simulink model "single-phase half bridge-controlled rectifier with resistive load"  (R2022a)
settings: Solver=VariableStepAuto  StartTime=0.0  StopTime=1  RelTol=1e-3
libraries: spsCurrentMeasurementLib x2, spsDiodeLib x2, spsSeriesRLCBranchLib x2, spsThyristorLib x2, spsVoltageMeasurementLib x2, spsACVoltageSourceLib x1, spspowerguiLib x1
settings Model: Creator=Joy  LastModifiedBy=Joy
settings SolverCC: AlgebraicLoopSolver=TrustRegion
settings DataIOCC: ReturnWorkspaceOutputs=off
settings RTWCC: DLArmComputeVersion=19.05

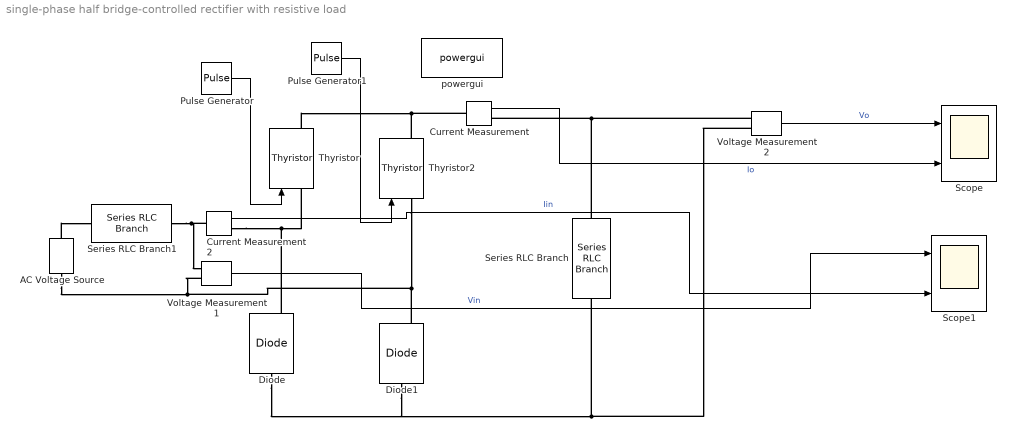
== system single-phase half bridge-controlled rectifier with resistive load ==
  AC Voltage Source : spsACVoltageSourceLib/AC Voltage Source  Amplitude=424.26  Phase=0  Frequency=60  SampleTime=0  Measurements=None  BusType=swing  Pref=10e3  Qref=0  Qmin=-inf  Qmax=+inf
  Current Measurement : spsCurrentMeasurementLib/Current Measurement  PhasorSimulation=off  OutputType=Complex  PSBequivalent=0
  Current Measurement2 : spsCurrentMeasurementLib/Current Measurement  PhasorSimulation=off  OutputType=Complex  PSBequivalent=0
  Diode : spsDiodeLib/Diode  Ron=0.001  Lon=0  Vf=0.8  IC=0  UseSnubber=0  Rs=500  Cs=250e-9  Measurements=on
  Diode1 : spsDiodeLib/Diode  Ron=0.001  Lon=0  Vf=0.8  IC=0  UseSnubber=0  Rs=500  Cs=250e-9  Measurements=on
  Pulse Generator : DiscretePulseGenerator  PulseType=Time based  Period=0.0167  PulseWidth=5  PhaseDelay=(1/60)*(30/360)
  Pulse Generator1 : DiscretePulseGenerator  PulseType=Time based  Period=0.0167  PulseWidth=5  PhaseDelay=(1/60)*(210/360)
  Scope : Scope  NumInputPorts=2
  Scope1 : Scope  NumInputPorts=2
  Series RLC Branch : spsSeriesRLCBranchLib/Series RLC Branch  LConnTagsString=__new0  RConnTagsString=__new0  BranchType=R  Resistance=20  Inductance=1e-3  SetiL0=off  InitialCurrent=0  Capacitance=1e-6  Setx0=off  InitialVoltage=0  Measurements=None
  Series RLC Branch1 : spsSeriesRLCBranchLib/Series RLC Branch  LConnTagsString=__new0  RConnTagsString=__new0  BranchType=L  Resistance=20  Inductance=1e-3  SetiL0=off  InitialCurrent=0  Capacitance=1e-6  Setx0=off  InitialVoltage=0  Measurements=None
  Thyristor : spsThyristorLib/Thyristor  Ron=0.001  Lon=0  Vf=0.8  IC=0  Rs=500  Cs=250e-9  Measurements=on
  Thyristor2 : spsThyristorLib/Thyristor  Ron=0.001  Lon=0  Vf=0.8  IC=0  Rs=500  Cs=250e-9  Measurements=on
  Voltage Measurement1 : spsVoltageMeasurementLib/Voltage Measurement  PhasorSimulation=off  OutputType=Complex  PSBequivalent=0
  Voltage Measurement2 : spsVoltageMeasurementLib/Voltage Measurement  PhasorSimulation=off  OutputType=Complex  PSBequivalent=0
  powergui : spspowerguiLib/powergui  Priority=1  SimulationMode=Continuous  SampleTime=50e-6  frequency=60  Iterations=50  frequencyindice=60  Pbase=100e6  ErrMax=1e-4  UnitsV=kV  UnitsW=MW  buscounter=0  FunctionMessages=off  echomessages=off  EnableUseOfTLC=off  CurrentSourceSwitches=off  DisableSnubberDevices=off  DisableRonSwitches=off  DisableVfSwitches=off  DisplayEquations=off  AutomaticDiscreteSolvers=off  SolverType=Tustin/Backward Euler (TBE)  Interpol=off  ExternalGateDelay=off  methode=off  Ts=100  x0status=blocks  SPID=on  SwTol=0  HookPort=off  NonlinearTolerance=1e-4  nMaxIteration=100  ContinueOnMaxIteration=off  RestoreLinks=warning  ResistiveCurrentMeasurement=off  Frange=[0:2:500]  Ylog=off  Xlog=on  ShowGrid=off  save=off  variable=ZData  structure=0  ZoomFFT=off  StartTime=0.0  cycles=1  DisplayStyle=1  fundamental=60  FreqAxis=off  MaxFrequency=1000  frequencyindicesteady=1  RmsSteady=1  display=off
  wires:
  Voltage Measurement2/1 -> Scope/1  "Vo"
  Current Measurement/1 -> Scope/2  "Io"
  Voltage Measurement1/1 -> Scope1/1  "Vin"
  Current Measurement2/1 -> Scope1/2  "Iin"
  Pulse Generator/1 -> Thyristor/1
  Pulse Generator1/1 -> Thyristor2/1
  connections:
  Current Measurement/LConn1 -- Thyristor/RConn1 -- Thyristor2/RConn1
  Series RLC Branch/LConn1 -- Voltage Measurement2/LConn1 -- Current Measurement/RConn1
  Current Measurement2/LConn1 -- Voltage Measurement1/LConn1 -- Series RLC Branch1/RConn1
  Thyristor2/LConn1 -- Diode1/RConn1 -- Voltage Measurement1/LConn2 -- AC Voltage Source/LConn1
  Current Measurement2/RConn1 -- Diode/RConn1 -- Thyristor/LConn1
  AC Voltage Source/RConn1 -- Series RLC Branch1/LConn1
  Voltage Measurement2/LConn2 -- Diode1/LConn1 -- Diode/LConn1 -- Series RLC Branch/RConn1
